simulink model "D3"  (R2017b)
settings: Solver=VariableStepAuto  StartTime=0.0  StopTime=700  RelTol=1e-3
libraries: simulink x3
settings Model: Creator=frank  LastModifiedBy=frank
settings SolverCC: ZeroCrossAlgorithm=Adaptive

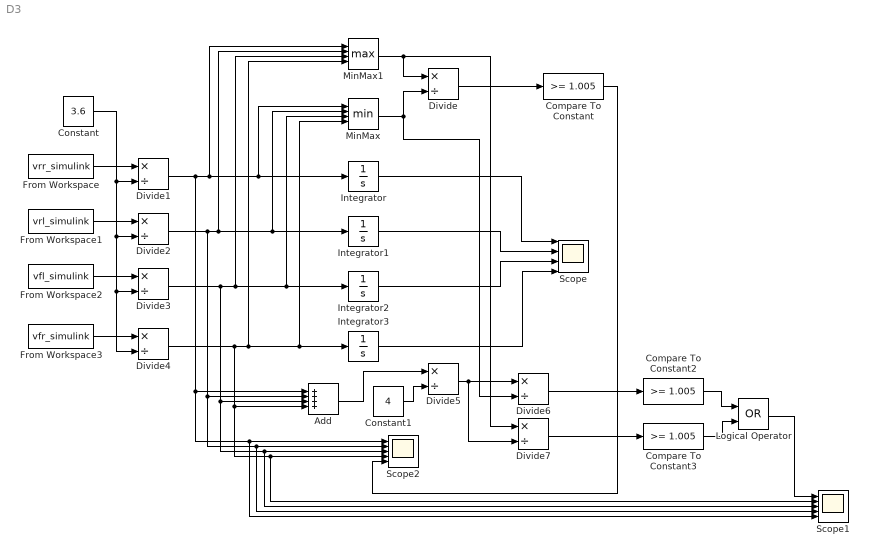
== system D3 ==
  Add : Sum  Inputs=4
  Compare To Constant : simulink/Logic and Bit Operations/Compare To Constant  relop=>=  const=1.005  OutDataTypeStr=boolean
  Compare To Constant2 : simulink/Logic and Bit Operations/Compare To Constant  relop=>=  const=1.005  OutDataTypeStr=boolean
  Compare To Constant3 : simulink/Logic and Bit Operations/Compare To Constant  relop=>=  const=1.005  OutDataTypeStr=boolean
  Constant : Constant  Value=3.6
  Constant1 : Constant  Value=4
  Divide{,1..7} (8 alike) : Product  Inputs=*/
  From Workspace : FromWorkspace  VariableName=vrr_simulink  SampleTime=0
  From Workspace1 : FromWorkspace  VariableName=vrl_simulink  SampleTime=0
  From Workspace2 : FromWorkspace  VariableName=vfl_simulink  SampleTime=0
  From Workspace3 : FromWorkspace  VariableName=vfr_simulink  SampleTime=0
  Integrator{,1..3} (4 alike) : Integrator
  Logical Operator : Logic  Operator=OR  AllPortsSameDT=off  OutDataTypeStr=boolean
  MinMax : MinMax  Inputs=4
  MinMax1 : MinMax  Function=max  Inputs=4
  Scope : Scope  NumInputPorts=4
  Scope1 : Scope  NumInputPorts=5
  Scope2 : Scope  NumInputPorts=5
  wires:
  Integrator/1 -> Scope/1
  Integrator1/1 -> Scope/2
  Integrator3/1 -> Scope/4
  Integrator2/1 -> Scope/3
  From Workspace/1 -> Divide1/1
  Divide1/1 -> Add/1, Scope1/5, Scope2/1, MinMax1/1, MinMax/1, Integrator/1
  From Workspace1/1 -> Divide2/1
  Divide2/1 -> Add/2, Scope1/4, Scope2/2, MinMax1/2, MinMax/2, Integrator1/1
  From Workspace2/1 -> Divide3/1
  From Workspace3/1 -> Divide4/1
  Constant/1 -> Divide4/2, Divide3/2, Divide2/2, Divide1/2
  Divide3/1 -> Add/3, Scope1/3, Scope2/3, MinMax1/3, MinMax/3, Integrator2/1
  MinMax1/1 -> Divide7/1, Divide/1
  MinMax/1 -> Divide/2, Divide6/2
  Divide/1 -> Compare To Constant/1
  Compare To Constant/1 -> Scope2/5
  Add/1 -> Divide5/1
  Constant1/1 -> Divide5/2
  Divide5/1 -> Divide7/2, Divide6/1
  Divide6/1 -> Compare To Constant2/1
  Divide7/1 -> Compare To Constant3/1
  Divide4/1 -> Add/4, Scope2/4, Scope1/2, MinMax1/4, MinMax/4, Integrator3/1
  Compare To Constant2/1 -> Logical Operator/1
  Compare To Constant3/1 -> Logical Operator/2
  Logical Operator/1 -> Scope1/1
